simulink model "pla_sim"  (R2024a)
settings: Solver=ode45  StartTime=0.0  StopTime=inf  RelTol=1e-3  EnableMultiTasking=on
settings Model: Creator=nunkesser  LastModifiedBy=nunkesser
settings SolverCC: AlgebraicLoopSolver=TrustRegion
settings DataIOCC: LimitDataPoints=on  SaveFormat=Array  ReturnWorkspaceOutputs=off
settings OptimizationCC: LifeSpan=inf
settings DebuggingCC: SolverPrmCheckMsg=warning  UnconnectedInputMsg=warning  UnconnectedOutputMsg=warning  UnconnectedLineMsg=warning  SFUnexpectedBacktrackingDiag=warning  SFNoUnconditionalDefaultTransitionDiag=warning  SFExecutionAtInitializationDiag=none  ArithmeticOperatorsInVariantConditions=warning
settings HardwareCC: ProdBitPerPointer=32  ProdBitPerSizeT=32  ProdBitPerPtrDiffT=32  ProdLargestAtomicFloat=None  ProdIntDivRoundTo=Undefined  ProdEndianess=Unspecified  ProdWordSize=32  ProdHWDeviceType=32-bit Generic
settings ModelReferenceCC: PropagateSignalLabelsOutOfModel=off
settings SFSimCC: SimUseLocalCustomCode=off  CustomCodeUndefinedFunction=UseInterfaceOnly
settings RTWCC: RTWUseLocalCustomCode=off  GPUComputeCapability=3.5
settings CodeAppCC: StateflowObjectComments=on
settings GRTTargetCC: TargetLangStandard=C89/C90 (ANSI)
settings ConfigComp: CovMetricSettings=dw  CovSaveCumulativeToWorkspaceVar=on  CovSaveSingleToWorkspaceVar=on  CovExternalEMLEnable=off  CovSFcnEnable=off

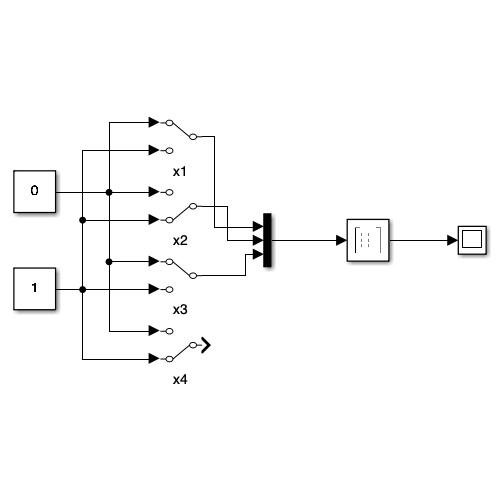
[thumbnail: Simulink's stored preview of the top-level diagram]
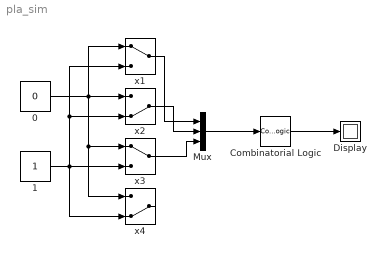
== system pla_sim ==
  0 : Constant  Value=0  OutDataTypeStr=boolean
  1 : Constant  OutDataTypeStr=boolean
  Combinatorial Logic : CombinatorialLogic  TruthTable=[0;1;1;0;1;0;0;1]
  Display : Display
  Mux : Mux  Inputs=3
  x1 : ManualSwitch
  x2 : ManualSwitch  CurrentSetting=0
  x3 : ManualSwitch
  x4 : ManualSwitch  CurrentSetting=0
  wires:
  0/1 -> x4/1, x3/1, x2/1, x1/1
  1/1 -> x4/2, x2/2, x1/2, x3/2
  x1/1 -> Mux/1
  x2/1 -> Mux/2
  x3/1 -> Mux/3
  Mux/1 -> Combinatorial Logic/1
  Combinatorial Logic/1 -> Display/1
